simulink model "test_model"  (R2020b)
settings: Solver=FixedStepAuto  StartTime=0.0  StopTime=[18;]  FixedStep=[0.01;]  RelTol=1e-3
settings Model: Creator=beave  LastModifiedBy=beave

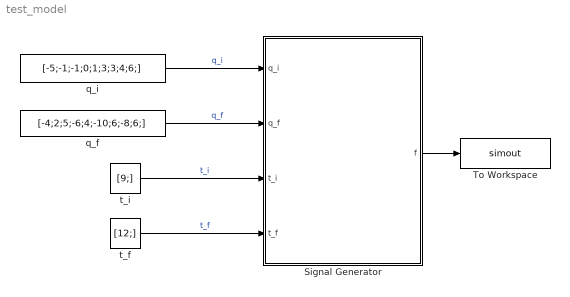
== system test_model ==
  Signal Generator : Subsystem
  To Workspace : ToWorkspace  VariableName=simout  SaveFormat=Timeseries  SampleTime=-1
  q_f : Constant  Value=[-4;2;5;-6;4;-10;6;-8;6;]
  q_i : Constant  Value=[-5;-1;-1;0;1;3;3;4;6;]
  t_f : Constant  Value=[12;]
  t_i : Constant  Value=[9;]
  wires:
  q_i/1 -> Signal Generator/1(q_i)  "q_i"
  q_f/1 -> Signal Generator/2(q_f)  "q_f"
  t_i/1 -> Signal Generator/3(t_i)  "t_i"
  t_f/1 -> Signal Generator/4(t_f)  "t_f"
  Signal Generator/1(f) -> To Workspace/1

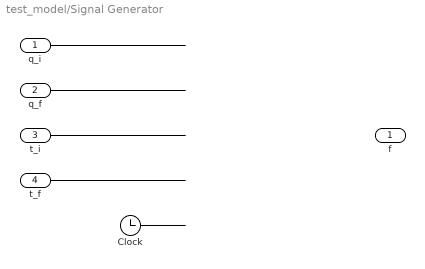
== system test_model/Signal Generator ==
  q_i : Inport
  q_f : Inport  Port=2
  t_i : Inport  Port=3
  t_f : Inport  Port=4
  Clock : Clock
  f : Outport
  wires:
  q_i/1 -> ?
  q_f/1 -> ?
  t_i/1 -> ?
  t_f/1 -> ?
  Clock/1 -> ?
  ? -> f/1
